simulink model "maain"  (Simulink 7.5)
settings: Solver=ode45  StartTime=0.0  StopTime=0.1  RelTol=1e-3
undefined symbols (not defined in the file): DiscIntNeverNeededParam, Hydride, Metal, Nickel, Ts
libraries: elec_lib x216, powerlib x32, fl_lib x9, powerlib_extras x7, electricdrivelib x2, simulink x2, nesl_utility x2
(part 1 of 2)
settings Model: Creator=quad  LastModifiedBy=quad

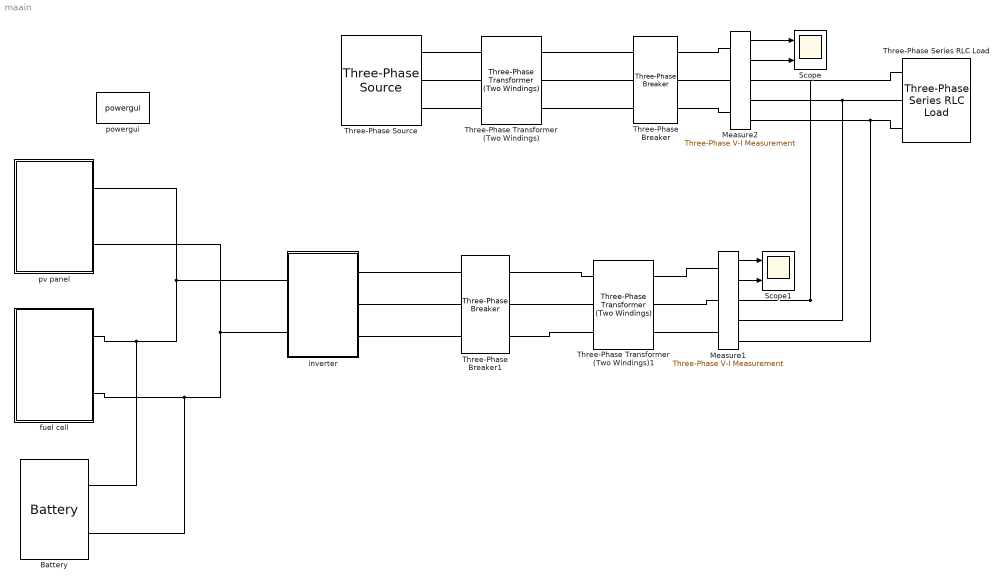
== system maain ==
  Battery : electricdrivelib/Extra Sources/Battery  DialogController=POWERSYS.PowerSysDialog  SystemSampleTime=-1  BatType=Nickel-Metal-Hydride  ShowDetailedParameters=off  NomV=1.2  NomQ=6.5  SOC=100  PresetModel=on  MaxQ=7  FullV=1.4136  Dis_rate=1.3  R=0.0018462  Normal_OP=6.25  expZone="[1.3017         1.3]"  Dis_Char=off  current=[6.5 13 32.5]  Units=Time  Batt_Tr=30
  Measure1 : powerlib/Measurements/Three-Phase V-I Measurement  DialogController=POWERSYS.PowerSysDialog  SystemSampleTime=-1  VoltageMeasurement=phase-to-ground  SetLabelV=off  LabelV=V1  Vpu=off  VpuLL=off  CurrentMeasurement=yes  SetLabelI=off  LabelI=I1  Ipu=off  Pbase=1e3  Vbase=380  OutputType=Magnitude  PhasorSimulation=off  PSBequivalent=0
      link override Model/VI/Ia: GotoTag=LibraryTag_Ia
      link override Model/VI/Ib: GotoTag=LibraryTag_Ib
      link override Model/VI/Ic: GotoTag=LibraryTag_Ic
      link override Model/VI/Va: GotoTag=LibraryTag_Va
      link override Model/VI/Vb: GotoTag=LibraryTag_Vb
      link override Model/VI/Vc: GotoTag=LibraryTag_Vc
  Measure2 : powerlib/Measurements/Three-Phase V-I Measurement  DialogController=POWERSYS.PowerSysDialog  SystemSampleTime=-1  VoltageMeasurement=phase-to-ground  SetLabelV=off  LabelV=V1  Vpu=off  VpuLL=off  CurrentMeasurement=yes  SetLabelI=off  LabelI=I1  Ipu=off  Pbase=1e3  Vbase=380  OutputType=Magnitude  PhasorSimulation=off  PSBequivalent=0
      link override Model/VI/Ia: GotoTag=LibraryTag_Ia
      link override Model/VI/Ib: GotoTag=LibraryTag_Ib
      link override Model/VI/Ic: GotoTag=LibraryTag_Ic
      link override Model/VI/Va: GotoTag=LibraryTag_Va
      link override Model/VI/Vb: GotoTag=LibraryTag_Vb
      link override Model/VI/Vc: GotoTag=LibraryTag_Vc
  Scope : Scope  NumInputPorts=2
      settings: YMin=-5000~-35  YMax=8000~55  SaveName=ScopeData4
  Scope1 : Scope  NumInputPorts=2
      settings: YMin=-0.35~-0.008  YMax=0.5~0.007  SaveName=ScopeData5
  Three-Phase Series RLC Load : powerlib/Elements/Three-Phase Series RLC Load  DialogController=POWERSYS.PowerSysDialog  PhysicalDomain=powersysdomain  SubClassName=unknown  LeftPortType=p1  RightPortType=p1  LConnTagsString=A|B|C  Configuration=Y (grounded)  NominalVoltage=380  NominalFrequency=50  ActivePower=1e3  InductivePower=0  CapacitivePower=0  Measurements=None
  Three-Phase Transformer (Two Windings) : powerlib/Elements/Three-Phase Transformer (Two Windings)  DialogController=POWERSYS.PowerSysDialog  SystemSampleTime=-1  Winding1Connection=Yg  UNITS=pu  NominalPower=[ 250e6 , 60 ]  Winding1=[ 735e3 , 0.002 , 0.08 ]  Winding2Connection=Yg  Winding2=[ 315e3 , 0.002 , 0.08 ]  SetSaturation=off  Rm=500  Lm=500  Saturation=[ 0,0 ; 0.0024,1.2 ; 1.0,1.52 ]  Hysteresis=off  DataFile='hysteresis'  SetInitialFlux=off  InitialFluxes=[ 0.8 , -0.8 , 0.7 ]  Measurements=None  MoreParameters=off  BreakLoop=off  DataType=off  TransfoNumber=1
  Three-Phase Transformer (Two Windings)1 : powerlib/Elements/Three-Phase Transformer (Two Windings)  DialogController=POWERSYS.PowerSysDialog  SystemSampleTime=-1  Winding1Connection=Yg  UNITS=pu  NominalPower=[ 250e6 , 60 ]  Winding1=[ 735e3 , 0.002 , 0.08 ]  Winding2Connection=Yg  Winding2=[ 315e3 , 0.002 , 0.08 ]  SetSaturation=off  Rm=500  Lm=500  Saturation=[ 0,0 ; 0.0024,1.2 ; 1.0,1.52 ]  Hysteresis=off  DataFile='hysteresis'  SetInitialFlux=off  InitialFluxes=[ 0.8 , -0.8 , 0.7 ]  Measurements=None  MoreParameters=off  BreakLoop=off  DataType=off  TransfoNumber=1
  Three-Phase Breaker : powerlib/Elements/Three-Phase Breaker  DialogController=POWERSYS.PowerSysDialog  SystemSampleTime=-1  InitialState=open  SwitchA=on  SwitchB=on  SwitchC=on  SwitchTimes="[4/60  10/60]"  External=off  BreakerResistance=0.001  SnubberResistance=1e6  SnubberCapacitance=inf  Measurements=None
  Three-Phase Breaker1 : powerlib/Elements/Three-Phase Breaker  DialogController=POWERSYS.PowerSysDialog  SystemSampleTime=-1  InitialState=closed  SwitchA=on  SwitchB=on  SwitchC=on  SwitchTimes="[4/60  10/60]"  External=off  BreakerResistance=0.001  SnubberResistance=1e6  SnubberCapacitance=inf  Measurements=None
  Three-Phase Source : powerlib/Electrical Sources/Three-Phase Source  DialogController=POWERSYS.PowerSysDialog  SystemSampleTime=-1  Voltage=25e3  PhaseAngle=0  Frequency=60  InternalConnection=Yg  SpecifyImpedance=on  Resistance=0.8929  Inductance=16.58e-3  ShortCircuitLevel=100e6  BaseVoltage=25e3  XRratio=7
  fuel cell : Subsystem
  inverter : Subsystem
  powergui : powerlib/powergui  Priority=1  SystemSampleTime=-1  SimulationMode=Continuous  SampleTime=50e-6  frequency=60  SPID=off  DisableSnubberDevices=off  DisableRonSwitches=off  DisableVfSwitches=off  SwTol=0  Interpol=off  frequencyindice=0  echomessages=off  HookPort=off  DisplayEquations=off  FunctionMessages=off  EnableUseOfTLC=off  x0status=blocks  RestoreLinks=warning  ResistiveCurrentMeasurement=off  Ylog=off  Xlog=on  ShowGrid=off  save=off  variable=ZData  ZoomFFT=off  StartTime=0.0  cycles=1  DisplayStyle=1  FreqAxis=off  MaxFrequency=1000  frequencyindicesteady=1  display=off  methode=off
  pv panel : Subsystem
  wires:
  Measure2/1 -> Scope/1
  Measure2/2 -> Scope/2
  Measure1/2 -> Scope1/2
  Measure1/1 -> Scope1/1
  connections:
  Three-Phase Source/RConn3 -- Three-Phase Transformer (Two Windings)/LConn3
  Three-Phase Source/RConn2 -- Three-Phase Transformer (Two Windings)/LConn2
  Three-Phase Source/RConn1 -- Three-Phase Transformer (Two Windings)/LConn1
  Measure1/RConn3 -- Three-Phase Series RLC Load/LConn3 -- Measure2/RConn3
  pv panel/RConn2 -- inverter/LConn2 -- fuel cell/RConn2 -- Battery/LConn2
  pv panel/RConn1 -- inverter/LConn1 -- fuel cell/RConn1 -- Battery/LConn1
  inverter/RConn1 -- Three-Phase Breaker1/LConn1
  inverter/RConn2 -- Three-Phase Breaker1/LConn2
  inverter/RConn3 -- Three-Phase Breaker1/LConn3
  Three-Phase Transformer (Two Windings)/RConn1 -- Three-Phase Breaker/LConn1
  Three-Phase Transformer (Two Windings)/RConn2 -- Three-Phase Breaker/LConn2
  Three-Phase Transformer (Two Windings)/RConn3 -- Three-Phase Breaker/LConn3
  Three-Phase Breaker/RConn1 -- Measure2/LConn1
  Three-Phase Breaker/RConn2 -- Measure2/LConn2
  Three-Phase Breaker/RConn3 -- Measure2/LConn3
  Measure1/RConn2 -- Three-Phase Series RLC Load/LConn2 -- Measure2/RConn2
  Measure1/RConn1 -- Three-Phase Series RLC Load/LConn1 -- Measure2/RConn1
  Three-Phase Breaker1/RConn1 -- Three-Phase Transformer (Two Windings)1/LConn1
  Three-Phase Breaker1/RConn2 -- Three-Phase Transformer (Two Windings)1/LConn2
  Three-Phase Breaker1/RConn3 -- Three-Phase Transformer (Two Windings)1/LConn3
  Three-Phase Transformer (Two Windings)1/RConn1 -- Measure1/LConn1
  Three-Phase Transformer (Two Windings)1/RConn2 -- Measure1/LConn2
  Three-Phase Transformer (Two Windings)1/RConn3 -- Measure1/LConn3

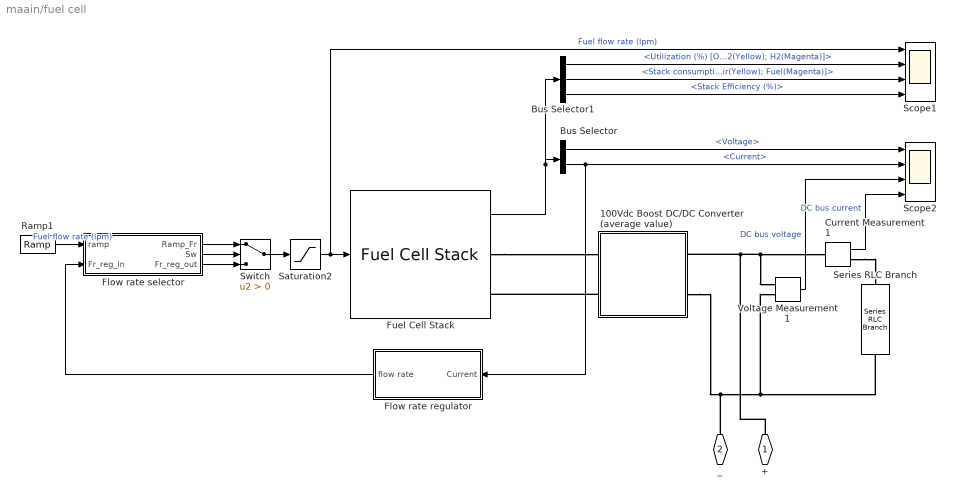
== system maain/fuel cell ==
  100Vdc Boost DC/DC Converter (average value) : Subsystem
  Bus Selector : BusSelector  OutputSignals=Voltage,Current
  Bus Selector1 : BusSelector  OutputSignals=Utilization (%) [O2(Yellow); H2(Magenta)],Stack consumption (lpm) [Air(Yellow); Fuel(Magenta)],Stack Efficiency (%)
  Current Measurement1 : powerlib/Measurements/Current Measurement  DialogController=POWERSYS.PowerSysDialog  SystemSampleTime=-1  PhasorSimulation=off  OutputType=Complex  PSBequivalent=0
  Flow rate regulator : Subsystem  mask{Nc=65, Uf_H2=99.56, T=65, Pf=1.5, x=99.95}
      mask prompts: Nc "Number of cells"; Uf_H2 "Nominal Hydrogen utilization (%)"; T "Operating temperature (Celsius)"; Pf "Fuel pressure (bar)"; x "H2 composition (%)"
  Flow rate selector : Subsystem
  Fuel Cell Stack : electricdrivelib/Extra Sources/Fuel Cell Stack  DialogController=POWERSYS.PowerSysDialog  SystemSampleTime=-1  PresetModel=PEMFC - 6 kW - 45 Vdc  FcType=Proton Exchange Membrane (PEM)  Detailed=Detailed  Eoc="[65  63]"  NomVI="[133.3            45]"  EndVI="[225   37]"  Nc=65  n=55  TOp=65  AirFr=300  SuppPress="[1.5           1]"  Comp="[99.95           21            1]"  plot_graph=off  ViewParam=off  SignX=off  SignY=off  FlowRateH2=on  FlowRateAir=off  SystemTemp=off  SystemPH2=off  SystemPAir=off  FCDyn=off  FC_tau=0  Peak_O2=80  V_Under=10
  Ramp1 : simulink/Sources/Ramp  SystemSampleTime=-1  slope=10  start=10  X0=0
  Saturation2 : Saturate  UpperLimit=85  LowerLimit=0  OutDataType=sfix(16)  OutScaling=2^0
  Scope1 : Scope  NumInputPorts=4
      settings: TimeRange=0.1  YMin=85~55~75~0.0443257  YMax=85~100~350~0.0443285  SaveName=ScopeData2
  Scope2 : Scope  NumInputPorts=4
      settings: TimeRange=0.1  YMin=0.0360995~249.771~1.44862~0.08196  YMax=0.036105~249.771~1.4488~0.081985  SaveName=ScopeData3
  Series RLC Branch : powerlib/Elements/Series RLC Branch  DialogController=POWERSYS.PowerSysDialog  PhysicalDomain=powersysdomain  SubClassName=unknown  LeftPortType=p1  RightPortType=p1  LConnTagsString=__new0  RConnTagsString=__new0  BranchType=RL  Resistance=100*100/6000  Inductance=100*100/6000  SetiL0=off  InitialCurrent=0  Capacitance=1e-6  Setx0=off  InitialVoltage=0  Measurements=None
  Switch : Switch  Criteria=u2 > Threshold  OutDataType=sfix(16)  OutScaling=2^0
  Voltage Measurement1 : powerlib/Measurements/Voltage Measurement  DialogController=POWERSYS.PowerSysDialog  SystemSampleTime=-1  PhasorSimulation=off  OutputType=Complex  PSBequivalent=0
  + : PMIOPort  Port=1  Side=Right
  _ : PMIOPort  Port=2  Side=Right
  wires:
  Fuel Cell Stack/1 -> Bus Selector/1, Bus Selector1/1
  Bus Selector/1 -> Scope2/1  "<Voltage>"
  Bus Selector/2 -> Scope2/2, Flow rate regulator/1(Current)  "<Current>"
  Voltage Measurement1/1 -> Scope2/3  "DC bus voltage"
  Current Measurement1/1 -> Scope2/4  "DC bus current"
  Bus Selector1/1 -> Scope1/2  "<Utilization (%) [O2(Yellow); H2(Magenta)]>"
  Bus Selector1/3 -> Scope1/4  "<Stack Efficiency (%)>"
  Bus Selector1/2 -> Scope1/3  "<Stack consumption (lpm) [Air(Yellow); Fuel(Magenta)]>"
  Ramp1/1 -> Flow rate selector/1(ramp)  "Fuel flow rate (lpm)"
  Switch/1 -> Saturation2/1
  Saturation2/1 -> Fuel Cell Stack/1, Scope1/1  "Fuel flow rate (lpm)"
  Flow rate selector/1(Ramp_Fr) -> Switch/1
  Flow rate selector/2(Sw) -> Switch/2
  Flow rate regulator/1(flow rate) -> Flow rate selector/2(Fr_reg_in)
  Flow rate selector/3(Fr_reg_out) -> Switch/3
  connections:
  100Vdc Boost DC/DC Converter (average value)/RConn2 -- Series RLC Branch/RConn1 -- Voltage Measurement1/LConn2 -- _/RConn1
  Voltage Measurement1/LConn1 -- Current Measurement1/LConn1 -- 100Vdc Boost DC/DC Converter (average value)/RConn1 -- +/RConn1
  100Vdc Boost DC/DC Converter (average value)/LConn2 -- Fuel Cell Stack/RConn2
  Current Measurement1/RConn1 -- Series RLC Branch/LConn1
  Fuel Cell Stack/RConn1 -- 100Vdc Boost DC/DC Converter (average value)/LConn1

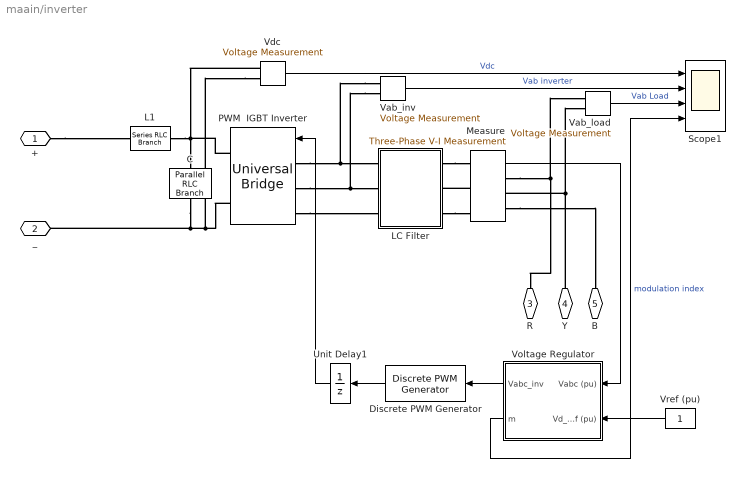
== system maain/inverter ==
  C : powerlib/Elements/Parallel RLC Branch  DialogController=POWERSYS.PowerSysDialog  PhysicalDomain=powersysdomain  SubClassName=unknown  LeftPortType=p1  RightPortType=p1  LConnTagsString=a  RConnTagsString=__new0  BranchType=RLC  Resistance=inf  Inductance=inf  SetiL0=off  InitialCurrent=0  Capacitance=5000e-06  Setx0=off  InitialVoltage=0  Measurements=None
  Discrete PWM Generator : powerlib_extras/Discrete  Control Blocks/Discrete PWM Generator  DialogController=POWERSYS.PowerSysDialog  SystemSampleTime=-1  GeneratorMode="3-arm  bridge (6 pulses)"  Fc=2000  Ts=Ts  Internal=off  mIndex=0.4  Freq=60  Phase=0
  L1 : powerlib/Elements/Series RLC Branch  DialogController=POWERSYS.PowerSysDialog  PhysicalDomain=powersysdomain  SubClassName=unknown  LeftPortType=p1  RightPortType=p1  LConnTagsString=__new0  RConnTagsString=__new0  BranchType=L  Resistance=1.0  Inductance=200e-6  SetiL0=off  InitialCurrent=0  Capacitance=1.0  Setx0=off  InitialVoltage=0  Measurements=None
  LC Filter : Subsystem
  Measure : powerlib/Measurements/Three-Phase V-I Measurement  DialogController=POWERSYS.PowerSysDialog  SystemSampleTime=-1  VoltageMeasurement=phase-to-ground  SetLabelV=off  LabelV=V1  Vpu=on  VpuLL=off  CurrentMeasurement=no  SetLabelI=off  LabelI=I1  Ipu=off  Pbase=1e3  Vbase=380  OutputType=Magnitude  PhasorSimulation=off  PSBequivalent=0
  PWM  IGBT Inverter : powerlib/Power Electronics/Universal Bridge  DialogController=POWERSYS.PowerSysDialog  SystemSampleTime=-1  Arms=3  SnubberResistance=5000  SnubberCapacitance=inf  Device=IGBT / Diodes  Ron=1e-3  Lon=0  ForwardVoltages="[  0.0  0.0  ]"  ForwardVoltage=.8  GTOparameters=[ 1e-6 ,1e-6 ]  IGBTparameters=[ 1e-6 , 2e-6 ]  Measurements=Device currents  Measurements_2=None  converterType=Rectifier
  Scope1 : Scope  NumInputPorts=4
      settings: TimeRange=0.1  YMin=1.725~-0.25~1.04~1  YMax=1.875~2~1.14~1  SaveName=psbbridges_str
  Unit Delay1 : UnitDelay  SampleTime=Ts
  Vab_inv : powerlib/Measurements/Voltage Measurement  Tag=PoWeRsYsTeMmEaSuReMeNt  DialogController=POWERSYS.PowerSysDialog  SystemSampleTime=-1  PhasorSimulation=off  OutputType=Magnitude  PSBequivalent=0
  Vab_load : powerlib/Measurements/Voltage Measurement  Tag=PoWeRsYsTeMmEaSuReMeNt  DialogController=POWERSYS.PowerSysDialog  SystemSampleTime=-1  PhasorSimulation=off  OutputType=Magnitude  PSBequivalent=0
  Vdc : powerlib/Measurements/Voltage Measurement  Tag=PoWeRsYsTeMmEaSuReMeNt  DialogController=POWERSYS.PowerSysDialog  SystemSampleTime=-1  PhasorSimulation=off  OutputType=Magnitude  PSBequivalent=0
  Voltage Regulator : Subsystem  mask( Voltage Regulator){Kp=0.4, Ki=500, Ts=Ts}
      mask prompts: Kp "Proportional gain  Kp:"; Ki "Integral gain Ki:"; Ts "Sample time (s) :"
  "Vref (pu) " : Constant  OutDataType=sfix(16)  OutScaling=2^0
  + : PMIOPort  Port=1  Side=Left
  _ : PMIOPort  Port=2  Side=Left
  R : PMIOPort  Port=3  Side=Right
  Y : PMIOPort  Port=4  Side=Right
  B : PMIOPort  Port=5  Side=Right
  wires:
  "Vref (pu) "/1 -> Voltage Regulator/2(Vd_ref (pu))
  Discrete PWM Generator/1 -> Unit Delay1/1
  Voltage Regulator/1(Vabc_inv) -> Discrete PWM Generator/1
  Voltage Regulator/2(m) -> Scope1/4  "modulation index"
  Vdc/1 -> Scope1/1  "Vdc"
  Vab_load/1 -> Scope1/3  "Vab Load"
  Vab_inv/1 -> Scope1/2  "Vab inverter"
  Unit Delay1/1 -> PWM  IGBT Inverter/1
  Measure/1 -> Voltage Regulator/1(Vabc (pu))
  connections:
  Vdc/LConn2 -- PWM  IGBT Inverter/RConn2 -- C/RConn1 -- _/RConn1
  PWM  IGBT Inverter/RConn1 -- Vdc/LConn1 -- C/LConn1 -- L1/RConn1
  Vab_inv/LConn2 -- PWM  IGBT Inverter/LConn2 -- LC Filter/LConn2
  Vab_inv/LConn1 -- PWM  IGBT Inverter/LConn1 -- LC Filter/LConn1
  Y/RConn1 -- Measure/RConn2 -- Vab_load/LConn2
  R/RConn1 -- Measure/RConn1 -- Vab_load/LConn1
  Measure/LConn2 -- LC Filter/RConn2
  Measure/RConn3 -- B/RConn1
  PWM  IGBT Inverter/LConn3 -- LC Filter/LConn3
  LC Filter/RConn1 -- Measure/LConn1
  LC Filter/RConn3 -- Measure/LConn3
  +/RConn1 -- L1/LConn1

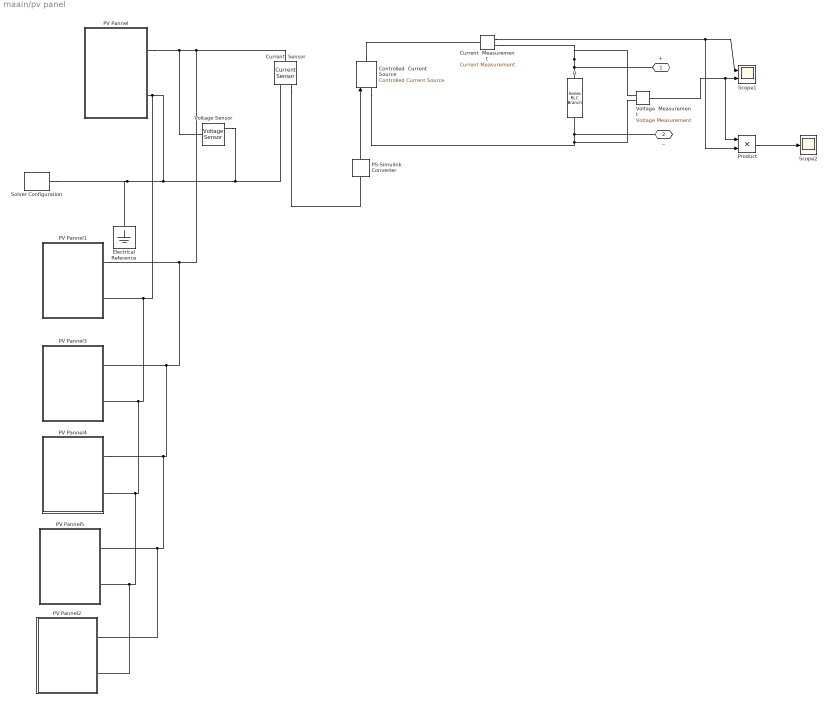
== system maain/pv panel ==
  " R " : powerlib/Elements/Series RLC Branch  DialogController=POWERSYS.PowerSysDialog  PhysicalDomain=powersysdomain  SubClassName=unknown  LeftPortType=p1  RightPortType=p1  LConnTagsString=__new0  RConnTagsString=__new0  BranchType=R  Resistance=10  Inductance=1e-3  SetiL0=off  InitialCurrent=0  Capacitance=1e-6  Setx0=off  InitialVoltage=0  Measurements=None
  Controlled  Current  Source : powerlib/Electrical Sources/Controlled Current Source  DialogController=POWERSYS.PowerSysDialog  SystemSampleTime=-1  Initialize=on  Source_Type=AC  Amplitude=0  Phase=0  Frequency=0  Measurements=None
  Current  Sensor : fl_lib/Electrical/Electrical Sensors/Current Sensor  DialogController=NetworkEngine.DynNeDlgSource  SystemSampleTime=-1  i1_Log=off  v1_Log=off  LocalVarNames=|i1|v1  LocalVarDescs=|i1|v1  LocalVarLogging=[0 0]
  Current  Measurement : powerlib/Measurements/Current Measurement  DialogController=POWERSYS.PowerSysDialog  SystemSampleTime=-1  PhasorSimulation=off  OutputType=Complex  PSBequivalent=0
  Electrical Reference : fl_lib/Electrical/Electrical Elements/Electrical Reference  DialogController=NetworkEngine.DynNeDlgSource  SystemSampleTime=-1  i_Log=off  LocalVarNames=|i  LocalVarDescs=|i  LocalVarLogging=0
  PS-Simulink Converter : nesl_utility/PS-Simulink Converter  DialogController=NetworkEngine.DynNeUtilDlgSource  SystemSampleTime=-1  PhysicalDomain=network_engine_domain  LeftPortType=input  RightPortType=output  SubClassName=ps_output  Unit=1  AffineConversion=off
  PV Pannel : Subsystem
  PV Pannel1 : Subsystem
  PV Pannel2 : Subsystem
  PV Pannel3 : Subsystem
  PV Pannel4 : Subsystem
  PV Pannel5 : Subsystem
  Product : Product  OutDataType=fixdt(1, 16)  OutScaling=2^0  RndMeth=Zero
  Scope1 : Scope  NumInputPorts=2
      settings: YMin=10.4699~1.63655  YMax=10.4699~1.6371
  Scope2 : Scope
      settings: YMin=17.1435  YMax=17.1465
  Solver Configuration : nesl_utility/Solver Configuration  DialogController=NetworkEngine.DynNeUtilDlgSource  SystemSampleTime=-1  PhysicalDomain=network_engine_domain  LeftPortType=input  RightPortType=generic  SubClassName=solver  Accelerate=off  Profile=off  ResidualTolerance=1e-9  MaxNonlinIter=3  MaxModeIter=2  DoFixedCost=off  UseLocalSampling=off  DoDC=off  LinearAlgebra=Sparse  LocalSolverSampleTime=.001  LocalSolverChoice=NE_BACKWARD_EULER_ADVANCER  UseLocalSolver=off
  Voltage  Measurement : powerlib/Measurements/Voltage Measurement  DialogController=POWERSYS.PowerSysDialog  SystemSampleTime=-1  PhasorSimulation=off  OutputType=Complex  PSBequivalent=0
  Voltage Sensor : fl_lib/Electrical/Electrical Sensors/Voltage Sensor  DialogController=NetworkEngine.DynNeDlgSource  SystemSampleTime=-1  i1_Log=off  v1_Log=off  LocalVarNames=|i1|v1  LocalVarDescs=|i1|v1  LocalVarLogging=[0 0]
  + : PMIOPort  Port=1  Side=Right
  _ : PMIOPort  Port=2  Side=Right
  wires:
  PS-Simulink Converter/1 -> Controlled  Current  Source/1
  Current  Measurement/1 -> Scope1/1, Product/2
  Voltage  Measurement/1 -> Product/1, Scope1/2
  Product/1 -> Scope2/1
  connections:
  PV Pannel3/LConn1 -- PV Pannel1/LConn1 -- Current  Sensor/LConn1 -- PV Pannel/LConn1 -- Voltage Sensor/LConn1 -- PV Pannel5/LConn1 -- PV Pannel2/LConn1 -- PV Pannel4/LConn1
  PV Pannel3/LConn2 -- Solver Configuration/RConn1 -- Electrical Reference/LConn1 -- Current  Sensor/RConn2 -- Voltage Sensor/RConn2 -- PV Pannel/LConn2 -- PV Pannel1/LConn2 -- PV Pannel5/LConn2 -- PV Pannel2/LConn2 -- PV Pannel4/LConn2
  Voltage  Measurement/LConn2 -- Controlled  Current  Source/LConn1 -- " R "/RConn1 -- _/RConn1
  Voltage  Measurement/LConn1 -- Current  Measurement/RConn1 -- " R "/LConn1 -- +/RConn1
  Current  Measurement/LConn1 -- Controlled  Current  Source/RConn1
  Current  Sensor/RConn1 -- PS-Simulink Converter/LConn1

== system maain/fuel cell/100Vdc Boost DC/DC Converter (average value) ==
  CBus : powerlib/Elements/Series RLC Branch  DialogController=POWERSYS.PowerSysDialog  PhysicalDomain=powersysdomain  SubClassName=unknown  LeftPortType=p1  RightPortType=p1  LConnTagsString=__new0  RConnTagsString=__new0  BranchType=RC  Resistance=0.2  Inductance=1e-3  SetiL0=off  InitialCurrent=0  Capacitance=7500e-6  Setx0=on  InitialVoltage=100  Measurements=None
  Chopper : Subsystem  mask(SPSdrives Converter){SnubberResistance=10e3, SnubberCapacitance=inf, Ron=1e-3, ForwardVoltages=[1.3,1.3], IGBTParameters=[0,0], converterType=Inverter}
      mask prompts: SnubberResistance "Snubber resistance Rs (Ohms):"; SnubberCapacitance "Snubber capacitance Cs (F):"; Ron "Ron (Ohms):"; ForwardVoltages "Forward voltages [Device Vf(V), Diode Vd (V)]"; IGBTParameters "[Tf(s), Tt(s)]:"; converterType "Converter type:"
      mask help: This model implements an average-value buck converter."Duty Cycle" contains the duty cycle of the internal IGBT device.
      mask StyleString: edit,edit,edit,edit,edit,popup(Rectifier|Inverter)
      mask Display: plot(0,0,100,100,[39 39 23.8],[71 28 28],[44 56 49.6 56 52.8 56 61 61],[39.2 33.6 32.8 33.6 40.8 33.6 30 12.4],[44 44 44 61 61],[28 71 60 66.4 90],[75 67 83 75 67 83 75 75],[54 42 42 54 54 54 54 66],[61 75 75],[24 24 42],[75 75 61],[66,76,76])
  Constant : Constant  Value=100  OutDataType=sfix(16)  OutScaling=2^0
  Current controller DISCRETE1 : Subsystem  mask(PI controller){Kp=0.0005, Ki=0.15, Ts=1e-3}
      mask prompts: Kp "Proportional gain (Kp)"; Ki "Integral gain (Ki)"; Ts "Sample time (s) :"
      mask help: Proportional-Integral Speed Controller
      mask Display: plot(0,0,100,100,[35,35,65],[70,30,30],[35,65],[45,60])
  Duty Cycles : Subsystem
  L : powerlib/Elements/Series RLC Branch  DialogController=POWERSYS.PowerSysDialog  PhysicalDomain=powersysdomain  SubClassName=unknown  LeftPortType=p1  RightPortType=p1  LConnTagsString=__new0  RConnTagsString=__new0  BranchType=L  Resistance=0.3  Inductance=500e-6  SetiL0=off  InitialCurrent=0  Capacitance=100e-6  Setx0=off  InitialVoltage=0  Measurements=None
  Transfer Fcn : TransferFcn  Denominator=[0.001 1]
  Voltage Measurement : powerlib/Measurements/Voltage Measurement  DialogController=POWERSYS.PowerSysDialog  SystemSampleTime=-1  PhasorSimulation=off  OutputType=Complex  PSBequivalent=0
  + : PMIOPort  Tag=PMCPort  Port=1  Side=Right
  - : PMIOPort  Tag=PMCPort  Port=2  Side=Right
  + FC : PMIOPort  Tag=PMCPort  Port=3  Side=Left
  - FC : PMIOPort  Tag=PMCPort  Port=4  Side=Left
  wires:
  Constant/1 -> Current controller DISCRETE1/2(Uref)
  Voltage Measurement/1 -> Transfer Fcn/1
  Duty Cycles/1(dc) -> Chopper/1(Duty Cycle)
  Transfer Fcn/1 -> Current controller DISCRETE1/1(UBus)
  Current controller DISCRETE1/1(Ec) -> Duty Cycles/1(Ec)
  connections:
  - FC/RConn1 -- Voltage Measurement/LConn2 -- -/RConn1 -- CBus/RConn1 -- Chopper/LConn2
  Voltage Measurement/LConn1 -- +/RConn1 -- Chopper/LConn1 -- CBus/LConn1
  Chopper/RConn1 -- L/LConn1
  + FC/RConn1 -- L/RConn1

== system maain/fuel cell/Flow rate regulator ==
  Current : Inport
  Fcn1 : Fcn  Expr=60000*8.3145*(273+T)*Nc*u(1)/(2*96485*(Pf*101325)*Uf_H2/100*x/100)
  Saturation : Saturate  UpperLimit=inf  LowerLimit=1  OutDataType=sfix(16)  OutScaling=2^0
  flow rate : Outport
  wires:
  Fcn1/1 -> Saturation/1
  Current/1 -> Fcn1/1
  Saturation/1 -> flow rate/1

== system maain/fuel cell/Flow rate selector ==
  ramp : Inport
  Fr_reg_in : Inport  Port=2
  Add : Sum  OutDataType=sfix(16)  OutScaling=2^-10
  Clock : Clock
  Compare To Constant : simulink/Logic and Bit Operations/Compare To Constant  SystemSampleTime=-1  relop=>  const=10  LogicOutDataTypeMode=boolean
  Edge Detector : powerlib_extras/Control  Blocks/Edge Detector  DialogController=POWERSYS.PowerSysDialog  SystemSampleTime=-1  model=Rising  ic=0
  Sample & Hold : powerlib_extras/Control  Blocks/Sample & Hold  DialogController=POWERSYS.PowerSysDialog  SystemSampleTime=-1  ic=0
  Ramp_Fr : Outport
  Sw : Outport  Port=2
  Fr_reg_out : Outport  Port=3
  wires:
  Clock/1 -> Compare To Constant/1
  Compare To Constant/1 -> Edge Detector/1, Sw/1
  Edge Detector/1 -> Sample & Hold/2
  Sample & Hold/1 -> Add/2
  Fr_reg_in/1 -> Sample & Hold/1, Fr_reg_out/1
  ramp/1 -> Add/1
  Add/1 -> Ramp_Fr/1

== system maain/inverter/LC Filter ==
  "2 mH " : powerlib/Elements/Three-Phase Series RLC Branch  DialogController=POWERSYS.PowerSysDialog  PhysicalDomain=powersysdomain  SubClassName=unknown  LeftPortType=p1  RightPortType=p1  LConnTagsString=A|B|C  RConnTagsString=A|B|C  BranchType=L  Resistance=1.0  Inductance=2e-3  Capacitance=1.0  Measurements=None
  3 kvar : powerlib/Elements/Three-Phase Series RLC Load  DialogController=POWERSYS.PowerSysDialog  PhysicalDomain=powersysdomain  SubClassName=unknown  LeftPortType=p1  RightPortType=p1  LConnTagsString=A|B|C  Configuration=Y (grounded)  NominalVoltage=380  NominalFrequency=50  ActivePower=0  InductivePower=0  CapacitivePower=3e3  Measurements=None
  A : PMIOPort  Port=1  Side=Left
  B : PMIOPort  Port=2  Side=Left
  C : PMIOPort  Port=3  Side=Left
  "A " : PMIOPort  Port=4  Side=Right
  "B " : PMIOPort  Port=5  Side=Right
  "C " : PMIOPort  Port=6  Side=Right
  connections:
  B/RConn1 -- "2 mH "/LConn2
  A/RConn1 -- "2 mH "/LConn1
  C/RConn1 -- "2 mH "/LConn3
  "2 mH "/RConn1 -- "A "/RConn1 -- 3 kvar/LConn1
  "2 mH "/RConn2 -- "B "/RConn1 -- 3 kvar/LConn2
  "2 mH "/RConn3 -- "C "/RConn1 -- 3 kvar/LConn3

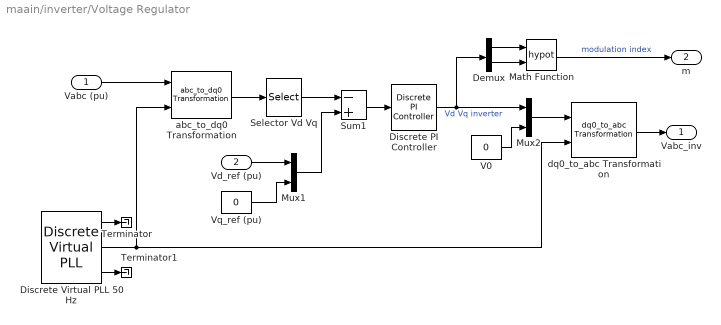
== system maain/inverter/Voltage Regulator ==
  Vabc (pu) : Inport  OutDataType=sfix(16)  OutScaling=2^0
  Vd_ref (pu) : Inport  Port=2  OutDataType=sfix(16)  OutScaling=2^0
  Demux : Demux  Outputs=2
  Discrete PI Controller : powerlib_extras/Discrete  Control Blocks/Discrete PI Controller  DialogController=POWERSYS.PowerSysDialog  SystemSampleTime=-1  Kp=Kp  Ki=Ki  Par_Limits=[1 -1]  Init=0  Ts=Ts
  Discrete Virtual PLL 50 Hz : powerlib_extras/Discrete  Control Blocks/Discrete Virtual PLL  DialogController=POWERSYS.PowerSysDialog  SystemSampleTime=-1  Freq=50  Phase=0  Ts=Ts
  Math Function : Math  Operator=hypot  OutDataType=sfix(16)  OutScaling=2^0  SaturateOnIntegerOverflow=on
  Mux1 : Mux  Inputs=2
  Mux2 : Mux  Inputs=2
  Selector Vd Vq : Selector  InputPortWidth=3  IndexOptions=Index vector (dialog)  Indices=[1 2]  OutputSizes=1
  Sum1 : Sum  Inputs=-+  OutDataType=sfix(16)  OutScaling=2^0  SaturateOnIntegerOverflow=on  InputSameDT=on  OutDataTypeStr=Inherit: Same as first input
  Terminator : Terminator
  Terminator1 : Terminator
  V0 : Constant  Value=0  OutDataType=sfix(16)  OutScaling=2^0
  Vq_ref (pu) : Constant  Value=0  OutDataType=sfix(16)  OutScaling=2^0
  abc_to_dq0 Transformation : powerlib_extras/Measurements/abc_to_dq0 Transformation  DialogController=POWERSYS.PowerSysDialog  SystemSampleTime=-1
  dq0_to_abc Transformation : powerlib_extras/Measurements/dq0_to_abc Transformation  DialogController=POWERSYS.PowerSysDialog  SystemSampleTime=-1
  Vabc_inv : Outport  OutDataType=sfix(16)  OutScaling=2^0
  m : Outport  Port=2  OutDataType=sfix(16)  OutScaling=2^0
  wires:
  abc_to_dq0 Transformation/1 -> Selector Vd Vq/1
  Vabc (pu)/1 -> abc_to_dq0 Transformation/1
  Selector Vd Vq/1 -> Sum1/1
  Sum1/1 -> Discrete PI Controller/1
  Mux2/1 -> dq0_to_abc Transformation/1
  V0/1 -> Mux2/2
  dq0_to_abc Transformation/1 -> Vabc_inv/1
  Discrete Virtual PLL 50 Hz/2 -> abc_to_dq0 Transformation/2, dq0_to_abc Transformation/2
  Vd_ref (pu)/1 -> Mux1/1
  Vq_ref (pu)/1 -> Mux1/2
  Mux1/1 -> Sum1/2
  Discrete Virtual PLL 50 Hz/1 -> Terminator/1
  Discrete Virtual PLL 50 Hz/3 -> Terminator1/1
  Discrete PI Controller/1 -> Demux/1, Mux2/1  "Vd Vq inverter"
  Demux/1 -> Math Function/1
  Demux/2 -> Math Function/2
  Math Function/1 -> m/1  "modulation index"

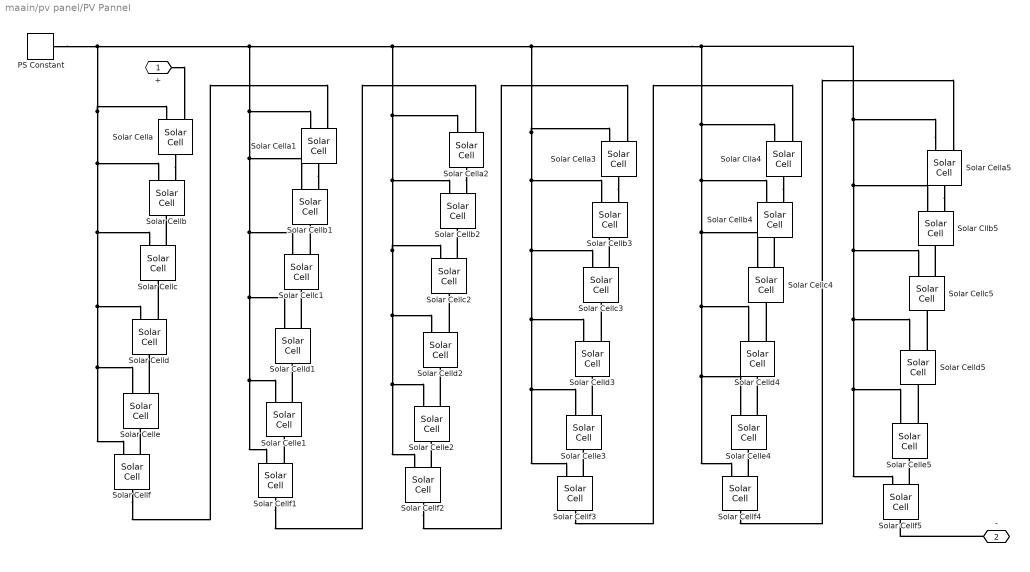
== system maain/pv panel/PV Pannel ==
  PS Constant : fl_lib/Physical Signals/Sources/PS Constant  DialogController=NetworkEngine.DynNeDlgSource  SystemSampleTime=-1  constant=687  LocalVarLogging=[]
  Solar Cella{,1..3,5} (5 alike) : elec_lib/Sources/Solar Cell  DialogController=NetworkEngine.DynNeDlgSource  SystemSampleTime=-1  prm=1  Isc=2.54 A  Voc=21.8 V  Is=1e-6 A  Is2=0 A  Iph=7.34 A  Ir0=1000 W/m^2  ec=1.6  N2=2  Rs=5.1e-3 Ohm  Rp=Inf Ohm  TIPH1=0.65e-3 1/K  EG=1.12 eV  TXIS1=3  TXIS2=3  TRS1=0  TRP1=0  TFIXED=25 C  Tmeas=25 C  LocalVarLogging=[]
  Solar Cellb{,1..4} (5 alike) : elec_lib/Sources/Solar Cell  DialogController=NetworkEngine.DynNeDlgSource  SystemSampleTime=-1  prm=1  Isc=2.54 A  Voc=21.8 V  Is=1e-6 A  Is2=0 A  Iph=7.34 A  Ir0=1000 W/m^2  ec=1.6  N2=2  Rs=5.1e-3 Ohm  Rp=Inf Ohm  TIPH1=0.65e-3 1/K  EG=1.12 eV  TXIS1=3  TXIS2=3  TRS1=0  TRP1=0  TFIXED=25 C  Tmeas=25 C  LocalVarLogging=[]
  Solar Cellc{,1..5} (6 alike) : elec_lib/Sources/Solar Cell  DialogController=NetworkEngine.DynNeDlgSource  SystemSampleTime=-1  prm=1  Isc=2.54 A  Voc=21.8 V  Is=1e-6 A  Is2=0 A  Iph=7.34 A  Ir0=1000 W/m^2  ec=1.6  N2=2  Rs=5.1e-3 Ohm  Rp=Inf Ohm  TIPH1=0.65e-3 1/K  EG=1.12 eV  TXIS1=3  TXIS2=3  TRS1=0  TRP1=0  TFIXED=25 C  Tmeas=25 C  LocalVarLogging=[]
  Solar Celld{,1..5} (6 alike) : elec_lib/Sources/Solar Cell  DialogController=NetworkEngine.DynNeDlgSource  SystemSampleTime=-1  prm=1  Isc=2.54 A  Voc=21.8 V  Is=1e-6 A  Is2=0 A  Iph=7.34 A  Ir0=1000 W/m^2  ec=1.6  N2=2  Rs=5.1e-3 Ohm  Rp=Inf Ohm  TIPH1=0.65e-3 1/K  EG=1.12 eV  TXIS1=3  TXIS2=3  TRS1=0  TRP1=0  TFIXED=25 C  Tmeas=25 C  LocalVarLogging=[]
  Solar Celle{,1..5} (6 alike) : elec_lib/Sources/Solar Cell  DialogController=NetworkEngine.DynNeDlgSource  SystemSampleTime=-1  prm=1  Isc=2.54 A  Voc=21.8 V  Is=1e-6 A  Is2=0 A  Iph=7.34 A  Ir0=1000 W/m^2  ec=1.6  N2=2  Rs=5.1e-3 Ohm  Rp=Inf Ohm  TIPH1=0.65e-3 1/K  EG=1.12 eV  TXIS1=3  TXIS2=3  TRS1=0  TRP1=0  TFIXED=25 C  Tmeas=25 C  LocalVarLogging=[]
  Solar Cellf{,1..5} (6 alike) : elec_lib/Sources/Solar Cell  DialogController=NetworkEngine.DynNeDlgSource  SystemSampleTime=-1  prm=1  Isc=2.54 A  Voc=21.8 V  Is=1e-6 A  Is2=0 A  Iph=7.34 A  Ir0=1000 W/m^2  ec=1.6  N2=2  Rs=5.1e-3 Ohm  Rp=Inf Ohm  TIPH1=0.65e-3 1/K  EG=1.12 eV  TXIS1=3  TXIS2=3  TRS1=0  TRP1=0  TFIXED=25 C  Tmeas=25 C  LocalVarLogging=[]
  Solar Clla4 : elec_lib/Sources/Solar Cell  DialogController=NetworkEngine.DynNeDlgSource  SystemSampleTime=-1  prm=1  Isc=2.54 A  Voc=21.8 V  Is=1e-6 A  Is2=0 A  Iph=7.34 A  Ir0=1000 W/m^2  ec=1.6  N2=2  Rs=5.1e-3 Ohm  Rp=Inf Ohm  TIPH1=0.65e-3 1/K  EG=1.12 eV  TXIS1=3  TXIS2=3  TRS1=0  TRP1=0  TFIXED=25 C  Tmeas=25 C  LocalVarLogging=[]
  Solar Cllb5 : elec_lib/Sources/Solar Cell  DialogController=NetworkEngine.DynNeDlgSource  SystemSampleTime=-1  prm=1  Isc=2.54 A  Voc=21.8 V  Is=1e-6 A  Is2=0 A  Iph=7.34 A  Ir0=1000 W/m^2  ec=1.6  N2=2  Rs=5.1e-3 Ohm  Rp=Inf Ohm  TIPH1=0.65e-3 1/K  EG=1.12 eV  TXIS1=3  TXIS2=3  TRS1=0  TRP1=0  TFIXED=25 C  Tmeas=25 C  LocalVarLogging=[]
  + : PMIOPort  Port=1  Side=Left
  - : PMIOPort  Port=2  Side=Left
  connections:
  Solar Cella/RConn1 -- Solar Cellb/LConn2
  Solar Cellc/LConn2 -- Solar Cellb/RConn1
  Solar Celld/LConn2 -- Solar Cellc/RConn1
  Solar Celle/LConn2 -- Solar Celld/RConn1
  Solar Cellf/LConn2 -- Solar Celle/RConn1
  Solar Cella1/RConn1 -- Solar Cellb1/LConn2
  Solar Cellc1/LConn2 -- Solar Cellb1/RConn1
  Solar Celld1/LConn2 -- Solar Cellc1/RConn1
  Solar Celle1/LConn2 -- Solar Celld1/RConn1
  Solar Cellf1/LConn2 -- Solar Celle1/RConn1
  Solar Cella2/RConn1 -- Solar Cellb2/LConn2
  Solar Cellc2/LConn2 -- Solar Cellb2/RConn1
  Solar Celld2/LConn2 -- Solar Cellc2/RConn1
  Solar Celle2/LConn2 -- Solar Celld2/RConn1
  Solar Cellf2/LConn2 -- Solar Celle2/RConn1
  Solar Cella3/RConn1 -- Solar Cellb3/LConn2
  Solar Cellc3/LConn2 -- Solar Cellb3/RConn1
  Solar Celld3/LConn2 -- Solar Cellc3/RConn1
  Solar Celle3/LConn2 -- Solar Celld3/RConn1
  Solar Cellf3/LConn2 -- Solar Celle3/RConn1
  Solar Clla4/RConn1 -- Solar Cellb4/LConn2
  Solar Cellc4/LConn2 -- Solar Cellb4/RConn1
  Solar Celld4/LConn2 -- Solar Cellc4/RConn1
  Solar Celle4/LConn2 -- Solar Celld4/RConn1
  Solar Cellf4/LConn2 -- Solar Celle4/RConn1
  Solar Cella5/RConn1 -- Solar Cllb5/LConn2
  Solar Cellc5/LConn2 -- Solar Cllb5/RConn1
  Solar Celld5/LConn2 -- Solar Cellc5/RConn1
  Solar Celle5/LConn2 -- Solar Celld5/RConn1
  Solar Cellf5/LConn2 -- Solar Celle5/RConn1
  Solar Cellf/RConn1 -- Solar Cella1/LConn2
  Solar Cellf1/RConn1 -- Solar Cella2/LConn2
  Solar Cellf2/RConn1 -- Solar Cella3/LConn2
  Solar Cellf3/RConn1 -- Solar Clla4/LConn2
  Solar Cellf4/RConn1 -- Solar Cella5/LConn2
  Solar Cella5/LConn1 -- Solar Cllb5/LConn1 -- Solar Cellc5/LConn1 -- Solar Celld5/LConn1 -- Solar Cellf5/LConn1 -- Solar Celle5/LConn1 -- PS Constant/RConn1 -- Solar Cellf/LConn1 -- Solar Celle/LConn1 -- Solar Celld/LConn1 -- Solar Cellc/LConn1 -- Solar Cellb/LConn1 -- Solar Cella/LConn1 -- Solar Cellf1/LConn1 -- Solar Celle1/LConn1 -- Solar Celld1/LConn1 -- Solar Cellc1/LConn1 -- Solar Cellb1/LConn1 -- Solar Cella1/LConn1 -- Solar Cella2/LConn1 -- Solar Cellb2/LConn1 -- Solar Cellc2/LConn1 -- Solar Celld2/LConn1 -- Solar Cellf2/LConn1 -- Solar Celle2/LConn1 -- Solar Cellf3/LConn1 -- Solar Celle3/LConn1 -- Solar Celld3/LConn1 -- Solar Cellc3/LConn1 -- Solar Cellb3/LConn1 -- Solar Cella3/LConn1 -- Solar Cellf4/LConn1 -- Solar Celle4/LConn1 -- Solar Celld4/LConn1 -- Solar Cellc4/LConn1 -- Solar Cellb4/LConn1 -- Solar Clla4/LConn1
  +/RConn1 -- Solar Cella/LConn2
  -/RConn1 -- Solar Cellf5/RConn1

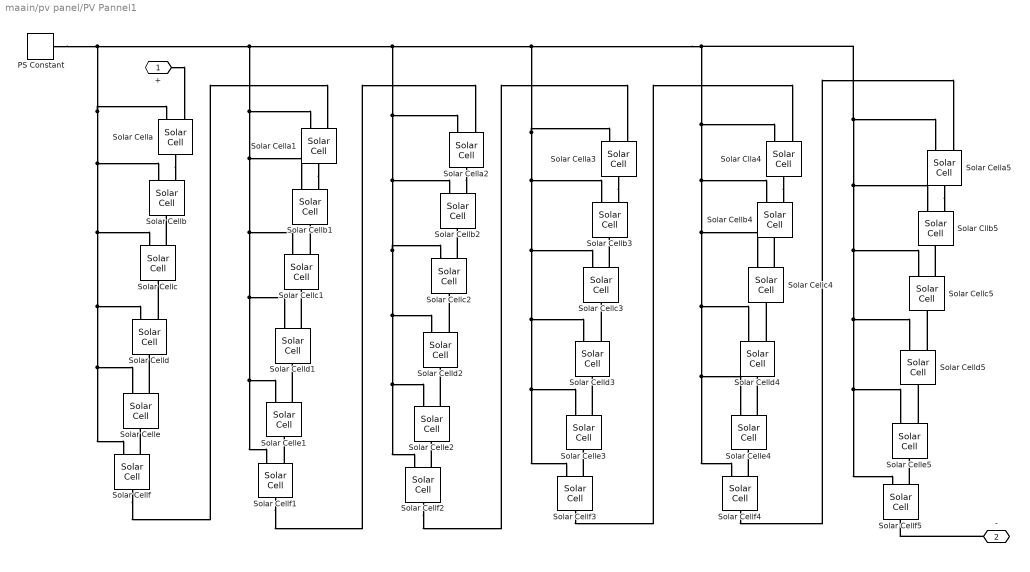
== system maain/pv panel/PV Pannel1 ==
  PS Constant : fl_lib/Physical Signals/Sources/PS Constant  DialogController=NetworkEngine.DynNeDlgSource  SystemSampleTime=-1  constant=687  LocalVarLogging=[]
  Solar Cella{,1..3,5} (5 alike) : elec_lib/Sources/Solar Cell  DialogController=NetworkEngine.DynNeDlgSource  SystemSampleTime=-1  prm=1  Isc=2.54 A  Voc=21.8 V  Is=1e-6 A  Is2=0 A  Iph=7.34 A  Ir0=1000 W/m^2  ec=1.6  N2=2  Rs=5.1e-3 Ohm  Rp=Inf Ohm  TIPH1=0.65e-3 1/K  EG=1.12 eV  TXIS1=3  TXIS2=3  TRS1=0  TRP1=0  TFIXED=25 C  Tmeas=25 C  LocalVarLogging=[]
  Solar Cellb{,1..4} (5 alike) : elec_lib/Sources/Solar Cell  DialogController=NetworkEngine.DynNeDlgSource  SystemSampleTime=-1  prm=1  Isc=2.54 A  Voc=21.8 V  Is=1e-6 A  Is2=0 A  Iph=7.34 A  Ir0=1000 W/m^2  ec=1.6  N2=2  Rs=5.1e-3 Ohm  Rp=Inf Ohm  TIPH1=0.65e-3 1/K  EG=1.12 eV  TXIS1=3  TXIS2=3  TRS1=0  TRP1=0  TFIXED=25 C  Tmeas=25 C  LocalVarLogging=[]
  Solar Cellc{,1..5} (6 alike) : elec_lib/Sources/Solar Cell  DialogController=NetworkEngine.DynNeDlgSource  SystemSampleTime=-1  prm=1  Isc=2.54 A  Voc=21.8 V  Is=1e-6 A  Is2=0 A  Iph=7.34 A  Ir0=1000 W/m^2  ec=1.6  N2=2  Rs=5.1e-3 Ohm  Rp=Inf Ohm  TIPH1=0.65e-3 1/K  EG=1.12 eV  TXIS1=3  TXIS2=3  TRS1=0  TRP1=0  TFIXED=25 C  Tmeas=25 C  LocalVarLogging=[]
  Solar Celld{,1..5} (6 alike) : elec_lib/Sources/Solar Cell  DialogController=NetworkEngine.DynNeDlgSource  SystemSampleTime=-1  prm=1  Isc=2.54 A  Voc=21.8 V  Is=1e-6 A  Is2=0 A  Iph=7.34 A  Ir0=1000 W/m^2  ec=1.6  N2=2  Rs=5.1e-3 Ohm  Rp=Inf Ohm  TIPH1=0.65e-3 1/K  EG=1.12 eV  TXIS1=3  TXIS2=3  TRS1=0  TRP1=0  TFIXED=25 C  Tmeas=25 C  LocalVarLogging=[]
  Solar Celle{,1..5} (6 alike) : elec_lib/Sources/Solar Cell  DialogController=NetworkEngine.DynNeDlgSource  SystemSampleTime=-1  prm=1  Isc=2.54 A  Voc=21.8 V  Is=1e-6 A  Is2=0 A  Iph=7.34 A  Ir0=1000 W/m^2  ec=1.6  N2=2  Rs=5.1e-3 Ohm  Rp=Inf Ohm  TIPH1=0.65e-3 1/K  EG=1.12 eV  TXIS1=3  TXIS2=3  TRS1=0  TRP1=0  TFIXED=25 C  Tmeas=25 C  LocalVarLogging=[]
  Solar Cellf{,1..5} (6 alike) : elec_lib/Sources/Solar Cell  DialogController=NetworkEngine.DynNeDlgSource  SystemSampleTime=-1  prm=1  Isc=2.54 A  Voc=21.8 V  Is=1e-6 A  Is2=0 A  Iph=7.34 A  Ir0=1000 W/m^2  ec=1.6  N2=2  Rs=5.1e-3 Ohm  Rp=Inf Ohm  TIPH1=0.65e-3 1/K  EG=1.12 eV  TXIS1=3  TXIS2=3  TRS1=0  TRP1=0  TFIXED=25 C  Tmeas=25 C  LocalVarLogging=[]
  Solar Clla4 : elec_lib/Sources/Solar Cell  DialogController=NetworkEngine.DynNeDlgSource  SystemSampleTime=-1  prm=1  Isc=2.54 A  Voc=21.8 V  Is=1e-6 A  Is2=0 A  Iph=7.34 A  Ir0=1000 W/m^2  ec=1.6  N2=2  Rs=5.1e-3 Ohm  Rp=Inf Ohm  TIPH1=0.65e-3 1/K  EG=1.12 eV  TXIS1=3  TXIS2=3  TRS1=0  TRP1=0  TFIXED=25 C  Tmeas=25 C  LocalVarLogging=[]
  Solar Cllb5 : elec_lib/Sources/Solar Cell  DialogController=NetworkEngine.DynNeDlgSource  SystemSampleTime=-1  prm=1  Isc=2.54 A  Voc=21.8 V  Is=1e-6 A  Is2=0 A  Iph=7.34 A  Ir0=1000 W/m^2  ec=1.6  N2=2  Rs=5.1e-3 Ohm  Rp=Inf Ohm  TIPH1=0.65e-3 1/K  EG=1.12 eV  TXIS1=3  TXIS2=3  TRS1=0  TRP1=0  TFIXED=25 C  Tmeas=25 C  LocalVarLogging=[]
  + : PMIOPort  Port=1  Side=Left
  - : PMIOPort  Port=2  Side=Left
  connections:
  -/RConn1 -- Solar Cellf5/RConn1
  +/RConn1 -- Solar Cella/LConn2
  Solar Cella3/LConn1 -- Solar Cellb3/LConn1 -- Solar Cellc3/LConn1 -- Solar Celld3/LConn1 -- Solar Celle3/LConn1 -- Solar Cellf3/LConn1 -- Solar Celle2/LConn1 -- Solar Cellf2/LConn1 -- Solar Celld2/LConn1 -- Solar Cellc2/LConn1 -- Solar Cellb2/LConn1 -- Solar Cella2/LConn1 -- Solar Cella1/LConn1 -- Solar Cellb1/LConn1 -- Solar Cellc1/LConn1 -- Solar Celld1/LConn1 -- Solar Celle1/LConn1 -- Solar Cellf1/LConn1 -- Solar Cella/LConn1 -- Solar Cellb/LConn1 -- Solar Cellc/LConn1 -- Solar Celld/LConn1 -- Solar Celle/LConn1 -- Solar Cellf/LConn1 -- PS Constant/RConn1 -- Solar Celle5/LConn1 -- Solar Cellf5/LConn1 -- Solar Celld5/LConn1 -- Solar Cellc5/LConn1 -- Solar Cllb5/LConn1 -- Solar Cella5/LConn1 -- Solar Clla4/LConn1 -- Solar Cellb4/LConn1 -- Solar Cellc4/LConn1 -- Solar Celld4/LConn1 -- Solar Celle4/LConn1 -- Solar Cellf4/LConn1
  Solar Cellf4/RConn1 -- Solar Cella5/LConn2
  Solar Cellf3/RConn1 -- Solar Clla4/LConn2
  Solar Cellf2/RConn1 -- Solar Cella3/LConn2
  Solar Cellf1/RConn1 -- Solar Cella2/LConn2
  Solar Cellf/RConn1 -- Solar Cella1/LConn2
  Solar Cellf5/LConn2 -- Solar Celle5/RConn1
  Solar Celle5/LConn2 -- Solar Celld5/RConn1
  Solar Celld5/LConn2 -- Solar Cellc5/RConn1
  Solar Cellc5/LConn2 -- Solar Cllb5/RConn1
  Solar Cella5/RConn1 -- Solar Cllb5/LConn2
  Solar Cellf4/LConn2 -- Solar Celle4/RConn1
  Solar Celle4/LConn2 -- Solar Celld4/RConn1
  Solar Celld4/LConn2 -- Solar Cellc4/RConn1
  Solar Cellc4/LConn2 -- Solar Cellb4/RConn1
  Solar Clla4/RConn1 -- Solar Cellb4/LConn2
  Solar Cellf3/LConn2 -- Solar Celle3/RConn1
  Solar Celle3/LConn2 -- Solar Celld3/RConn1
  Solar Celld3/LConn2 -- Solar Cellc3/RConn1
  Solar Cellc3/LConn2 -- Solar Cellb3/RConn1
  Solar Cella3/RConn1 -- Solar Cellb3/LConn2
  Solar Cellf2/LConn2 -- Solar Celle2/RConn1
  Solar Celle2/LConn2 -- Solar Celld2/RConn1
  Solar Celld2/LConn2 -- Solar Cellc2/RConn1
  Solar Cellc2/LConn2 -- Solar Cellb2/RConn1
  Solar Cella2/RConn1 -- Solar Cellb2/LConn2
  Solar Cellf1/LConn2 -- Solar Celle1/RConn1
  Solar Celle1/LConn2 -- Solar Celld1/RConn1
  Solar Celld1/LConn2 -- Solar Cellc1/RConn1
  Solar Cellc1/LConn2 -- Solar Cellb1/RConn1
  Solar Cella1/RConn1 -- Solar Cellb1/LConn2
  Solar Cellf/LConn2 -- Solar Celle/RConn1
  Solar Celle/LConn2 -- Solar Celld/RConn1
  Solar Celld/LConn2 -- Solar Cellc/RConn1
  Solar Cellc/LConn2 -- Solar Cellb/RConn1
  Solar Cella/RConn1 -- Solar Cellb/LConn2

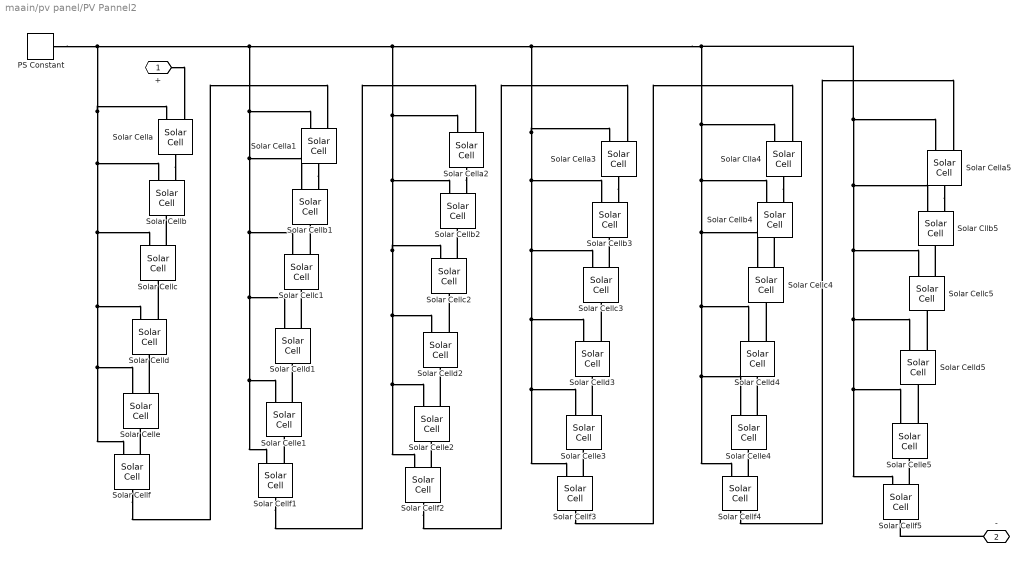
== system maain/pv panel/PV Pannel2 ==
  PS Constant : fl_lib/Physical Signals/Sources/PS Constant  DialogController=NetworkEngine.DynNeDlgSource  SystemSampleTime=-1  constant=687  LocalVarLogging=[]
  Solar Cella{,1..3,5} (5 alike) : elec_lib/Sources/Solar Cell  DialogController=NetworkEngine.DynNeDlgSource  SystemSampleTime=-1  prm=1  Isc=2.54 A  Voc=21.8 V  Is=1e-6 A  Is2=0 A  Iph=7.34 A  Ir0=1000 W/m^2  ec=1.6  N2=2  Rs=5.1e-3 Ohm  Rp=Inf Ohm  TIPH1=0.65e-3 1/K  EG=1.12 eV  TXIS1=3  TXIS2=3  TRS1=0  TRP1=0  TFIXED=25 C  Tmeas=25 C  LocalVarLogging=[]
  Solar Cellb{,1..4} (5 alike) : elec_lib/Sources/Solar Cell  DialogController=NetworkEngine.DynNeDlgSource  SystemSampleTime=-1  prm=1  Isc=2.54 A  Voc=21.8 V  Is=1e-6 A  Is2=0 A  Iph=7.34 A  Ir0=1000 W/m^2  ec=1.6  N2=2  Rs=5.1e-3 Ohm  Rp=Inf Ohm  TIPH1=0.65e-3 1/K  EG=1.12 eV  TXIS1=3  TXIS2=3  TRS1=0  TRP1=0  TFIXED=25 C  Tmeas=25 C  LocalVarLogging=[]
  Solar Cellc{,1..5} (6 alike) : elec_lib/Sources/Solar Cell  DialogController=NetworkEngine.DynNeDlgSource  SystemSampleTime=-1  prm=1  Isc=2.54 A  Voc=21.8 V  Is=1e-6 A  Is2=0 A  Iph=7.34 A  Ir0=1000 W/m^2  ec=1.6  N2=2  Rs=5.1e-3 Ohm  Rp=Inf Ohm  TIPH1=0.65e-3 1/K  EG=1.12 eV  TXIS1=3  TXIS2=3  TRS1=0  TRP1=0  TFIXED=25 C  Tmeas=25 C  LocalVarLogging=[]
  Solar Celld{,1..5} (6 alike) : elec_lib/Sources/Solar Cell  DialogController=NetworkEngine.DynNeDlgSource  SystemSampleTime=-1  prm=1  Isc=2.54 A  Voc=21.8 V  Is=1e-6 A  Is2=0 A  Iph=7.34 A  Ir0=1000 W/m^2  ec=1.6  N2=2  Rs=5.1e-3 Ohm  Rp=Inf Ohm  TIPH1=0.65e-3 1/K  EG=1.12 eV  TXIS1=3  TXIS2=3  TRS1=0  TRP1=0  TFIXED=25 C  Tmeas=25 C  LocalVarLogging=[]
  Solar Celle{,1..5} (6 alike) : elec_lib/Sources/Solar Cell  DialogController=NetworkEngine.DynNeDlgSource  SystemSampleTime=-1  prm=1  Isc=2.54 A  Voc=21.8 V  Is=1e-6 A  Is2=0 A  Iph=7.34 A  Ir0=1000 W/m^2  ec=1.6  N2=2  Rs=5.1e-3 Ohm  Rp=Inf Ohm  TIPH1=0.65e-3 1/K  EG=1.12 eV  TXIS1=3  TXIS2=3  TRS1=0  TRP1=0  TFIXED=25 C  Tmeas=25 C  LocalVarLogging=[]
  Solar Cellf{,1..5} (6 alike) : elec_lib/Sources/Solar Cell  DialogController=NetworkEngine.DynNeDlgSource  SystemSampleTime=-1  prm=1  Isc=2.54 A  Voc=21.8 V  Is=1e-6 A  Is2=0 A  Iph=7.34 A  Ir0=1000 W/m^2  ec=1.6  N2=2  Rs=5.1e-3 Ohm  Rp=Inf Ohm  TIPH1=0.65e-3 1/K  EG=1.12 eV  TXIS1=3  TXIS2=3  TRS1=0  TRP1=0  TFIXED=25 C  Tmeas=25 C  LocalVarLogging=[]
  Solar Clla4 : elec_lib/Sources/Solar Cell  DialogController=NetworkEngine.DynNeDlgSource  SystemSampleTime=-1  prm=1  Isc=2.54 A  Voc=21.8 V  Is=1e-6 A  Is2=0 A  Iph=7.34 A  Ir0=1000 W/m^2  ec=1.6  N2=2  Rs=5.1e-3 Ohm  Rp=Inf Ohm  TIPH1=0.65e-3 1/K  EG=1.12 eV  TXIS1=3  TXIS2=3  TRS1=0  TRP1=0  TFIXED=25 C  Tmeas=25 C  LocalVarLogging=[]
  Solar Cllb5 : elec_lib/Sources/Solar Cell  DialogController=NetworkEngine.DynNeDlgSource  SystemSampleTime=-1  prm=1  Isc=2.54 A  Voc=21.8 V  Is=1e-6 A  Is2=0 A  Iph=7.34 A  Ir0=1000 W/m^2  ec=1.6  N2=2  Rs=5.1e-3 Ohm  Rp=Inf Ohm  TIPH1=0.65e-3 1/K  EG=1.12 eV  TXIS1=3  TXIS2=3  TRS1=0  TRP1=0  TFIXED=25 C  Tmeas=25 C  LocalVarLogging=[]
  + : PMIOPort  Port=1  Side=Left
  - : PMIOPort  Port=2  Side=Left
  connections:
  -/RConn1 -- Solar Cellf5/RConn1
  +/RConn1 -- Solar Cella/LConn2
  Solar Cella3/LConn1 -- Solar Cellb3/LConn1 -- Solar Cellc3/LConn1 -- Solar Celld3/LConn1 -- Solar Celle3/LConn1 -- Solar Cellf3/LConn1 -- Solar Celle2/LConn1 -- Solar Cellf2/LConn1 -- Solar Celld2/LConn1 -- Solar Cellc2/LConn1 -- Solar Cellb2/LConn1 -- Solar Cella2/LConn1 -- Solar Cella1/LConn1 -- Solar Cellb1/LConn1 -- Solar Cellc1/LConn1 -- Solar Celld1/LConn1 -- Solar Celle1/LConn1 -- Solar Cellf1/LConn1 -- Solar Cella/LConn1 -- Solar Cellb/LConn1 -- Solar Cellc/LConn1 -- Solar Celld/LConn1 -- Solar Celle/LConn1 -- Solar Cellf/LConn1 -- PS Constant/RConn1 -- Solar Celle5/LConn1 -- Solar Cellf5/LConn1 -- Solar Celld5/LConn1 -- Solar Cellc5/LConn1 -- Solar Cllb5/LConn1 -- Solar Cella5/LConn1 -- Solar Clla4/LConn1 -- Solar Cellb4/LConn1 -- Solar Cellc4/LConn1 -- Solar Celld4/LConn1 -- Solar Celle4/LConn1 -- Solar Cellf4/LConn1
  Solar Cellf4/RConn1 -- Solar Cella5/LConn2
  Solar Cellf3/RConn1 -- Solar Clla4/LConn2
  Solar Cellf2/RConn1 -- Solar Cella3/LConn2
  Solar Cellf1/RConn1 -- Solar Cella2/LConn2
  Solar Cellf/RConn1 -- Solar Cella1/LConn2
  Solar Cellf5/LConn2 -- Solar Celle5/RConn1
  Solar Celle5/LConn2 -- Solar Celld5/RConn1
  Solar Celld5/LConn2 -- Solar Cellc5/RConn1
  Solar Cellc5/LConn2 -- Solar Cllb5/RConn1
  Solar Cella5/RConn1 -- Solar Cllb5/LConn2
  Solar Cellf4/LConn2 -- Solar Celle4/RConn1
  Solar Celle4/LConn2 -- Solar Celld4/RConn1
  Solar Celld4/LConn2 -- Solar Cellc4/RConn1
  Solar Cellc4/LConn2 -- Solar Cellb4/RConn1
  Solar Clla4/RConn1 -- Solar Cellb4/LConn2
  Solar Cellf3/LConn2 -- Solar Celle3/RConn1
  Solar Celle3/LConn2 -- Solar Celld3/RConn1
  Solar Celld3/LConn2 -- Solar Cellc3/RConn1
  Solar Cellc3/LConn2 -- Solar Cellb3/RConn1
  Solar Cella3/RConn1 -- Solar Cellb3/LConn2
  Solar Cellf2/LConn2 -- Solar Celle2/RConn1
  Solar Celle2/LConn2 -- Solar Celld2/RConn1
  Solar Celld2/LConn2 -- Solar Cellc2/RConn1
  Solar Cellc2/LConn2 -- Solar Cellb2/RConn1
  Solar Cella2/RConn1 -- Solar Cellb2/LConn2
  Solar Cellf1/LConn2 -- Solar Celle1/RConn1
  Solar Celle1/LConn2 -- Solar Celld1/RConn1
  Solar Celld1/LConn2 -- Solar Cellc1/RConn1
  Solar Cellc1/LConn2 -- Solar Cellb1/RConn1
  Solar Cella1/RConn1 -- Solar Cellb1/LConn2
  Solar Cellf/LConn2 -- Solar Celle/RConn1
  Solar Celle/LConn2 -- Solar Celld/RConn1
  Solar Celld/LConn2 -- Solar Cellc/RConn1
  Solar Cellc/LConn2 -- Solar Cellb/RConn1
  Solar Cella/RConn1 -- Solar Cellb/LConn2

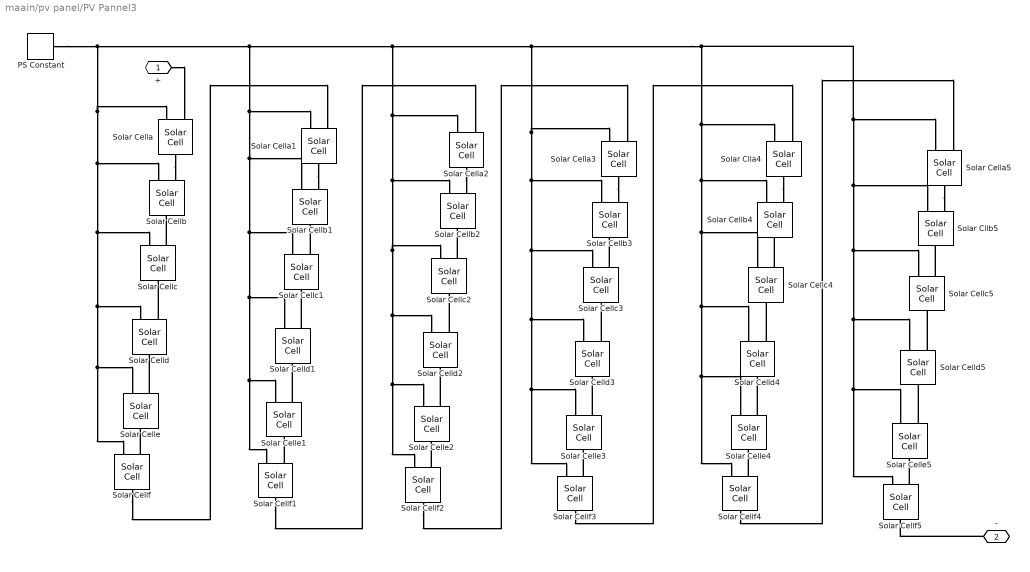
== system maain/pv panel/PV Pannel3 ==
  PS Constant : fl_lib/Physical Signals/Sources/PS Constant  DialogController=NetworkEngine.DynNeDlgSource  SystemSampleTime=-1  constant=687  LocalVarLogging=[]
  Solar Cella{,1..3,5} (5 alike) : elec_lib/Sources/Solar Cell  DialogController=NetworkEngine.DynNeDlgSource  SystemSampleTime=-1  prm=1  Isc=2.54 A  Voc=21.8 V  Is=1e-6 A  Is2=0 A  Iph=7.34 A  Ir0=1000 W/m^2  ec=1.6  N2=2  Rs=5.1e-3 Ohm  Rp=Inf Ohm  TIPH1=0.65e-3 1/K  EG=1.12 eV  TXIS1=3  TXIS2=3  TRS1=0  TRP1=0  TFIXED=25 C  Tmeas=25 C  LocalVarLogging=[]
  Solar Cellb{,1..4} (5 alike) : elec_lib/Sources/Solar Cell  DialogController=NetworkEngine.DynNeDlgSource  SystemSampleTime=-1  prm=1  Isc=2.54 A  Voc=21.8 V  Is=1e-6 A  Is2=0 A  Iph=7.34 A  Ir0=1000 W/m^2  ec=1.6  N2=2  Rs=5.1e-3 Ohm  Rp=Inf Ohm  TIPH1=0.65e-3 1/K  EG=1.12 eV  TXIS1=3  TXIS2=3  TRS1=0  TRP1=0  TFIXED=25 C  Tmeas=25 C  LocalVarLogging=[]
  Solar Cellc{,1..5} (6 alike) : elec_lib/Sources/Solar Cell  DialogController=NetworkEngine.DynNeDlgSource  SystemSampleTime=-1  prm=1  Isc=2.54 A  Voc=21.8 V  Is=1e-6 A  Is2=0 A  Iph=7.34 A  Ir0=1000 W/m^2  ec=1.6  N2=2  Rs=5.1e-3 Ohm  Rp=Inf Ohm  TIPH1=0.65e-3 1/K  EG=1.12 eV  TXIS1=3  TXIS2=3  TRS1=0  TRP1=0  TFIXED=25 C  Tmeas=25 C  LocalVarLogging=[]
  Solar Celld{,1..5} (6 alike) : elec_lib/Sources/Solar Cell  DialogController=NetworkEngine.DynNeDlgSource  SystemSampleTime=-1  prm=1  Isc=2.54 A  Voc=21.8 V  Is=1e-6 A  Is2=0 A  Iph=7.34 A  Ir0=1000 W/m^2  ec=1.6  N2=2  Rs=5.1e-3 Ohm  Rp=Inf Ohm  TIPH1=0.65e-3 1/K  EG=1.12 eV  TXIS1=3  TXIS2=3  TRS1=0  TRP1=0  TFIXED=25 C  Tmeas=25 C  LocalVarLogging=[]
  Solar Celle{,1..5} (6 alike) : elec_lib/Sources/Solar Cell  DialogController=NetworkEngine.DynNeDlgSource  SystemSampleTime=-1  prm=1  Isc=2.54 A  Voc=21.8 V  Is=1e-6 A  Is2=0 A  Iph=7.34 A  Ir0=1000 W/m^2  ec=1.6  N2=2  Rs=5.1e-3 Ohm  Rp=Inf Ohm  TIPH1=0.65e-3 1/K  EG=1.12 eV  TXIS1=3  TXIS2=3  TRS1=0  TRP1=0  TFIXED=25 C  Tmeas=25 C  LocalVarLogging=[]
  Solar Cellf{,1..5} (6 alike) : elec_lib/Sources/Solar Cell  DialogController=NetworkEngine.DynNeDlgSource  SystemSampleTime=-1  prm=1  Isc=2.54 A  Voc=21.8 V  Is=1e-6 A  Is2=0 A  Iph=7.34 A  Ir0=1000 W/m^2  ec=1.6  N2=2  Rs=5.1e-3 Ohm  Rp=Inf Ohm  TIPH1=0.65e-3 1/K  EG=1.12 eV  TXIS1=3  TXIS2=3  TRS1=0  TRP1=0  TFIXED=25 C  Tmeas=25 C  LocalVarLogging=[]
  Solar Clla4 : elec_lib/Sources/Solar Cell  DialogController=NetworkEngine.DynNeDlgSource  SystemSampleTime=-1  prm=1  Isc=2.54 A  Voc=21.8 V  Is=1e-6 A  Is2=0 A  Iph=7.34 A  Ir0=1000 W/m^2  ec=1.6  N2=2  Rs=5.1e-3 Ohm  Rp=Inf Ohm  TIPH1=0.65e-3 1/K  EG=1.12 eV  TXIS1=3  TXIS2=3  TRS1=0  TRP1=0  TFIXED=25 C  Tmeas=25 C  LocalVarLogging=[]
  Solar Cllb5 : elec_lib/Sources/Solar Cell  DialogController=NetworkEngine.DynNeDlgSource  SystemSampleTime=-1  prm=1  Isc=2.54 A  Voc=21.8 V  Is=1e-6 A  Is2=0 A  Iph=7.34 A  Ir0=1000 W/m^2  ec=1.6  N2=2  Rs=5.1e-3 Ohm  Rp=Inf Ohm  TIPH1=0.65e-3 1/K  EG=1.12 eV  TXIS1=3  TXIS2=3  TRS1=0  TRP1=0  TFIXED=25 C  Tmeas=25 C  LocalVarLogging=[]
  + : PMIOPort  Port=1  Side=Left
  - : PMIOPort  Port=2  Side=Left
  connections:
  -/RConn1 -- Solar Cellf5/RConn1
  +/RConn1 -- Solar Cella/LConn2
  Solar Cella3/LConn1 -- Solar Cellb3/LConn1 -- Solar Cellc3/LConn1 -- Solar Celld3/LConn1 -- Solar Celle3/LConn1 -- Solar Cellf3/LConn1 -- Solar Celle2/LConn1 -- Solar Cellf2/LConn1 -- Solar Celld2/LConn1 -- Solar Cellc2/LConn1 -- Solar Cellb2/LConn1 -- Solar Cella2/LConn1 -- Solar Cella1/LConn1 -- Solar Cellb1/LConn1 -- Solar Cellc1/LConn1 -- Solar Celld1/LConn1 -- Solar Celle1/LConn1 -- Solar Cellf1/LConn1 -- Solar Cella/LConn1 -- Solar Cellb/LConn1 -- Solar Cellc/LConn1 -- Solar Celld/LConn1 -- Solar Celle/LConn1 -- Solar Cellf/LConn1 -- PS Constant/RConn1 -- Solar Celle5/LConn1 -- Solar Cellf5/LConn1 -- Solar Celld5/LConn1 -- Solar Cellc5/LConn1 -- Solar Cllb5/LConn1 -- Solar Cella5/LConn1 -- Solar Clla4/LConn1 -- Solar Cellb4/LConn1 -- Solar Cellc4/LConn1 -- Solar Celld4/LConn1 -- Solar Celle4/LConn1 -- Solar Cellf4/LConn1
  Solar Cellf4/RConn1 -- Solar Cella5/LConn2
  Solar Cellf3/RConn1 -- Solar Clla4/LConn2
  Solar Cellf2/RConn1 -- Solar Cella3/LConn2
  Solar Cellf1/RConn1 -- Solar Cella2/LConn2
  Solar Cellf/RConn1 -- Solar Cella1/LConn2
  Solar Cellf5/LConn2 -- Solar Celle5/RConn1
  Solar Celle5/LConn2 -- Solar Celld5/RConn1
  Solar Celld5/LConn2 -- Solar Cellc5/RConn1
  Solar Cellc5/LConn2 -- Solar Cllb5/RConn1
  Solar Cella5/RConn1 -- Solar Cllb5/LConn2
  Solar Cellf4/LConn2 -- Solar Celle4/RConn1
  Solar Celle4/LConn2 -- Solar Celld4/RConn1
  Solar Celld4/LConn2 -- Solar Cellc4/RConn1
  Solar Cellc4/LConn2 -- Solar Cellb4/RConn1
  Solar Clla4/RConn1 -- Solar Cellb4/LConn2
  Solar Cellf3/LConn2 -- Solar Celle3/RConn1
  Solar Celle3/LConn2 -- Solar Celld3/RConn1
  Solar Celld3/LConn2 -- Solar Cellc3/RConn1
  Solar Cellc3/LConn2 -- Solar Cellb3/RConn1
  Solar Cella3/RConn1 -- Solar Cellb3/LConn2
  Solar Cellf2/LConn2 -- Solar Celle2/RConn1
  Solar Celle2/LConn2 -- Solar Celld2/RConn1
  Solar Celld2/LConn2 -- Solar Cellc2/RConn1
  Solar Cellc2/LConn2 -- Solar Cellb2/RConn1
  Solar Cella2/RConn1 -- Solar Cellb2/LConn2
  Solar Cellf1/LConn2 -- Solar Celle1/RConn1
  Solar Celle1/LConn2 -- Solar Celld1/RConn1
  Solar Celld1/LConn2 -- Solar Cellc1/RConn1
  Solar Cellc1/LConn2 -- Solar Cellb1/RConn1
  Solar Cella1/RConn1 -- Solar Cellb1/LConn2
  Solar Cellf/LConn2 -- Solar Celle/RConn1
  Solar Celle/LConn2 -- Solar Celld/RConn1
  Solar Celld/LConn2 -- Solar Cellc/RConn1
  Solar Cellc/LConn2 -- Solar Cellb/RConn1
  Solar Cella/RConn1 -- Solar Cellb/LConn2
